simulink model "PUMA_fuzzy_dis"  (Simulink 8.9)
settings: Solver=ode15s  StartTime=0  StopTime=5  MaxStep=0.02  RelTol=1e-3  EnableMultiTasking=on
undefined symbols (not defined in the file): sfunxyz
libraries: aerolibutil x17, simulink x4, Fuzzy_Type2_Lib x3
(part 3 of 3)

== system PUMA_fuzzy_dis/3-Link PUMA Robot-Block /K or I matrix = fct (tau: torque, B, C, G, dteta) /B matrix/b412/I14 ==
  AI14 actual I14 : Constant  Value=0.00164
  Sum4 : Sum  Inputs=|++
  UI14 uncertainty added to I14 +- 0.0009 max : Constant  Value=UI14
  I14 : Outport
  wires:
  AI14 actual I14/1 -> Sum4/1
  UI14 uncertainty added to I14 +- 0.0009 max/1 -> Sum4/2
  Sum4/1 -> I14/1

== system PUMA_fuzzy_dis/3-Link PUMA Robot-Block /K or I matrix = fct (tau: torque, B, C, G, dteta) /B matrix/b412/I19 ==
  AI19 actual I19 : Constant  Value=0.0003
  Sum4 : Sum  Inputs=|++
  UI19 uncertainty added to I19 +- 0.0003 max : Constant  Value=UI19
  I19 : Outport
  wires:
  AI19 actual I19/1 -> Sum4/1
  UI19 uncertainty added to I19 +- 0.0003 max/1 -> Sum4/2
  Sum4/1 -> I19/1

== system PUMA_fuzzy_dis/3-Link PUMA Robot-Block /K or I matrix = fct (tau: torque, B, C, G, dteta) /B matrix/b412/I20 ==
  AI20 actual I20 : Constant  Value=-0.000202
  Sum4 : Sum  Inputs=|++
  UI20 uncertainty added to I20 +- 0.0008 max : Constant  Value=UI20
  I20 : Outport
  wires:
  AI20 actual I20/1 -> Sum4/1
  UI20 uncertainty added to I20 +- 0.0008 max/1 -> Sum4/2
  Sum4/1 -> I20/1

== system PUMA_fuzzy_dis/3-Link PUMA Robot-Block /K or I matrix = fct (tau: torque, B, C, G, dteta) /B matrix/b413/I14 ==
  AI14 actual I14 : Constant  Value=0.00164
  Sum4 : Sum  Inputs=|++
  UI14 uncertainty added to I14 +- 0.0009 max : Constant  Value=UI14
  I14 : Outport
  wires:
  AI14 actual I14/1 -> Sum4/1
  UI14 uncertainty added to I14 +- 0.0009 max/1 -> Sum4/2
  Sum4/1 -> I14/1

== system PUMA_fuzzy_dis/3-Link PUMA Robot-Block /K or I matrix = fct (tau: torque, B, C, G, dteta) /B matrix/b413/I19 ==
  AI19 actual I19 : Constant  Value=0.0003
  Sum4 : Sum  Inputs=|++
  UI19 uncertainty added to I19 +- 0.0003 max : Constant  Value=UI19
  I19 : Outport
  wires:
  AI19 actual I19/1 -> Sum4/1
  UI19 uncertainty added to I19 +- 0.0003 max/1 -> Sum4/2
  Sum4/1 -> I19/1

== system PUMA_fuzzy_dis/3-Link PUMA Robot-Block /K or I matrix = fct (tau: torque, B, C, G, dteta) /B matrix/b413/I20 ==
  AI20 actual I20 : Constant  Value=-0.000202
  Sum4 : Sum  Inputs=|++
  UI20 uncertainty added to I20 +- 0.0008 max : Constant  Value=UI20
  I20 : Outport
  wires:
  AI20 actual I20/1 -> Sum4/1
  UI20 uncertainty added to I20 +- 0.0008 max/1 -> Sum4/2
  Sum4/1 -> I20/1

== system PUMA_fuzzy_dis/3-Link PUMA Robot-Block /K or I matrix = fct (tau: torque, B, C, G, dteta) /B matrix/b415/I17 ==
  AI17 actual I17 : Constant  Value=0.000642
  Sum4 : Sum  Inputs=|++
  UI17 uncertainty added to I17 +- 0.0003 max : Constant  Value=UI17
  I17 : Outport
  wires:
  AI17 actual I17/1 -> Sum4/1
  UI17 uncertainty added to I17 +- 0.0003 max/1 -> Sum4/2
  Sum4/1 -> I17/1

== system PUMA_fuzzy_dis/3-Link PUMA Robot-Block /K or I matrix = fct (tau: torque, B, C, G, dteta) /B matrix/b415/I20 ==
  AI20 actual I20 : Constant  Value=-0.000202
  Sum4 : Sum  Inputs=|++
  UI20 uncertainty added to I20 +- 0.0008 max : Constant  Value=UI20
  I20 : Outport
  wires:
  AI20 actual I20/1 -> Sum4/1
  UI20 uncertainty added to I20 +- 0.0008 max/1 -> Sum4/2
  Sum4/1 -> I20/1

== system PUMA_fuzzy_dis/3-Link PUMA Robot-Block /K or I matrix = fct (tau: torque, B, C, G, dteta) /B matrix/b514/I17 ==
  AI17 actual I17 : Constant  Value=0.000642
  Sum4 : Sum  Inputs=|++
  UI17 uncertainty added to I17 +- 0.0003 max : Constant  Value=UI17
  I17 : Outport
  wires:
  AI17 actual I17/1 -> Sum4/1
  UI17 uncertainty added to I17 +- 0.0003 max/1 -> Sum4/2
  Sum4/1 -> I17/1

== system PUMA_fuzzy_dis/3-Link PUMA Robot-Block /K or I matrix = fct (tau: torque, B, C, G, dteta) /B matrix/b514/I20 ==
  AI20 actual I20 : Constant  Value=-0.000202
  Sum4 : Sum  Inputs=|++
  UI20 uncertainty added to I20 +- 0.0008 max : Constant  Value=UI20
  I20 : Outport
  wires:
  AI20 actual I20/1 -> Sum4/1
  UI20 uncertainty added to I20 +- 0.0008 max/1 -> Sum4/2
  Sum4/1 -> I20/1

== system PUMA_fuzzy_dis/3-Link PUMA Robot-Block /K or I matrix = fct (tau: torque, B, C, G, dteta) /C matrix/c12/I13 ==
  AI13 actual I13 : Constant  Value=-0.00379
  Sum4 : Sum  Inputs=|++
  UI13 uncertainty added to I13 +- 0.0009 max : Constant  Value=UI13
  I13 : Outport
  wires:
  AI13 actual I13/1 -> Sum4/1
  UI13 uncertainty added to I13 +- 0.0009 max/1 -> Sum4/2
  Sum4/1 -> I13/1

== system PUMA_fuzzy_dis/3-Link PUMA Robot-Block /K or I matrix = fct (tau: torque, B, C, G, dteta) /C matrix/c12/I18 ==
  AI18 actual I18 : Constant  Value=0.000431
  Sum4 : Sum  Inputs=|++
  UI18 uncertainty added to I18 +- 0.0003 max : Constant  Value=UI18
  I18 : Outport
  wires:
  AI18 actual I18/1 -> Sum4/1
  UI18 uncertainty added to I18 +- 0.0003 max/1 -> Sum4/2
  Sum4/1 -> I18/1

== system PUMA_fuzzy_dis/3-Link PUMA Robot-Block /K or I matrix = fct (tau: torque, B, C, G, dteta) /C matrix/c12/I4 ==
  AI4 actual I4 : Constant  Value=0.69
  Sum4 : Sum  Inputs=|++
  UI4 uncertainty added to I4 +- 0.02 max : Constant  Value=UI4
  I4 : Outport
  wires:
  AI4 actual I4/1 -> Sum4/1
  UI4 uncertainty added to I4 +- 0.02 max/1 -> Sum4/2
  Sum4/1 -> I4/1

== system PUMA_fuzzy_dis/3-Link PUMA Robot-Block /K or I matrix = fct (tau: torque, B, C, G, dteta) /C matrix/c12/I8 ==
  AI8 actual I8 : Constant  Value=-0.134
  Sum4 : Sum  Inputs=|++
  UI8 uncertainty added to I8 +- 0.014 max : Constant  Value=UI8
  I8 : Outport
  wires:
  AI8 actual I8/1 -> Sum4/1
  UI8 uncertainty added to I8 +- 0.014 max/1 -> Sum4/2
  Sum4/1 -> I8/1

== system PUMA_fuzzy_dis/3-Link PUMA Robot-Block /K or I matrix = fct (tau: torque, B, C, G, dteta) /C matrix/c12/I9 ==
  AI9 actual I9 : Constant  Value=0.0238
  Sum4 : Sum  Inputs=|++
  UI9 uncertainty added to I9 +- 0.014 max : Constant  Value=UI9
  I9 : Outport
  wires:
  AI9 actual I9/1 -> Sum4/1
  UI9 uncertainty added to I9 +- 0.014 max/1 -> Sum4/2
  Sum4/1 -> I9/1

== system PUMA_fuzzy_dis/3-Link PUMA Robot-Block /K or I matrix = fct (tau: torque, B, C, G, dteta) /C matrix/c13/I13 ==
  AI13 actual I13 : Constant  Value=-0.00379
  Sum4 : Sum  Inputs=|++
  UI13 uncertainty added to I13 +- 0.0009 max : Constant  Value=UI13
  I13 : Outport
  wires:
  AI13 actual I13/1 -> Sum4/1
  UI13 uncertainty added to I13 +- 0.0009 max/1 -> Sum4/2
  Sum4/1 -> I13/1

== system PUMA_fuzzy_dis/3-Link PUMA Robot-Block /K or I matrix = fct (tau: torque, B, C, G, dteta) /C matrix/c13/I18 ==
  AI18 actual I18 : Constant  Value=0.000431
  Sum4 : Sum  Inputs=|++
  UI18 uncertainty added to I18 +- 0.0003 max : Constant  Value=UI18
  I18 : Outport
  wires:
  AI18 actual I18/1 -> Sum4/1
  UI18 uncertainty added to I18 +- 0.0003 max/1 -> Sum4/2
  Sum4/1 -> I18/1

== system PUMA_fuzzy_dis/3-Link PUMA Robot-Block /K or I matrix = fct (tau: torque, B, C, G, dteta) /C matrix/c13/I8 ==
  AI8 actual I8 : Constant  Value=-0.134
  Sum4 : Sum  Inputs=|++
  UI8 uncertainty added to I8 +- 0.014 max : Constant  Value=UI8
  I8 : Outport
  wires:
  AI8 actual I8/1 -> Sum4/1
  UI8 uncertainty added to I8 +- 0.014 max/1 -> Sum4/2
  Sum4/1 -> I8/1

== system PUMA_fuzzy_dis/3-Link PUMA Robot-Block /K or I matrix = fct (tau: torque, B, C, G, dteta) /C matrix/c21/I10 ==
  AI10 actual I10 : Constant  Value=-0.0213
  Sum4 : Sum  Inputs=|++
  UI10 uncertainty added to I10 +- 0.022 max : Constant  Value=UI10
  I10 : Outport
  wires:
  AI10 actual I10/1 -> Sum4/1
  UI10 uncertainty added to I10 +- 0.022 max/1 -> Sum4/2
  Sum4/1 -> I10/1

== system PUMA_fuzzy_dis/3-Link PUMA Robot-Block /K or I matrix = fct (tau: torque, B, C, G, dteta) /C matrix/c21/I11 ==
  AI11 actual I11 : Constant  Value=-0.0142
  Sum4 : Sum  Inputs=|++
  UI11 uncertainty added to I11 +- 0.007 max : Constant  Value=UI11
  I11 : Outport
  wires:
  AI11 actual I11/1 -> Sum4/1
  UI11 uncertainty added to I11 +- 0.007 max/1 -> Sum4/2
  Sum4/1 -> I11/1

== system PUMA_fuzzy_dis/3-Link PUMA Robot-Block /K or I matrix = fct (tau: torque, B, C, G, dteta) /C matrix/c21/I12 ==
  AI12 actual I12 : Constant  Value=-0.011
  Sum4 : Sum  Inputs=|++
  UI12 uncertainty added to I12 +- 0.0011 max : Constant  Value=UI12
  I12 : Outport
  wires:
  AI12 actual I12/1 -> Sum4/1
  UI12 uncertainty added to I12 +- 0.0011 max/1 -> Sum4/2
  Sum4/1 -> I12/1

== system PUMA_fuzzy_dis/3-Link PUMA Robot-Block /K or I matrix = fct (tau: torque, B, C, G, dteta) /C matrix/c21/I15 ==
  AI15 actual I15 : Constant  Value=0.00125
  Sum4 : Sum  Inputs=|++
  UI15 uncertainty added to I15 +- 0.0003 max : Constant  Value=UI15
  I15 : Outport
  wires:
  AI15 actual I15/1 -> Sum4/1
  UI15 uncertainty added to I15 +- 0.0003 max/1 -> Sum4/2
  Sum4/1 -> I15/1

== system PUMA_fuzzy_dis/3-Link PUMA Robot-Block /K or I matrix = fct (tau: torque, B, C, G, dteta) /C matrix/c21/I16 ==
  AI16 actual I16 : Constant  Value=0.00124
  Sum4 : Sum  Inputs=|++
  UI16 uncertainty added to I16 +- 0.0003 max : Constant  Value=UI16
  I16 : Outport
  wires:
  AI16 actual I16/1 -> Sum4/1
  UI16 uncertainty added to I16 +- 0.0003 max/1 -> Sum4/2
  Sum4/1 -> I16/1

== system PUMA_fuzzy_dis/3-Link PUMA Robot-Block /K or I matrix = fct (tau: torque, B, C, G, dteta) /C matrix/c21/I21 ==
  AI21 actual I21 : Constant  Value=-0.0001
  Sum4 : Sum  Inputs=|++
  UI21 uncertainty added to I21 +- 0.0006 max : Constant  Value=UI21
  I21 : Outport
  wires:
  AI21 actual I21/1 -> Sum4/1
  UI21 uncertainty added to I21 +- 0.0006 max/1 -> Sum4/2
  Sum4/1 -> I21/1

== system PUMA_fuzzy_dis/3-Link PUMA Robot-Block /K or I matrix = fct (tau: torque, B, C, G, dteta) /C matrix/c21/I22 ==
  AI22 actual I22 : Constant  Value=-0.000058
  Sum4 : Sum  Inputs=|++
  UI22 uncertainty added to I22 +- 0.000015 max : Constant  Value=UI22
  I22 : Outport
  wires:
  AI22 actual I22/1 -> Sum4/1
  UI22 uncertainty added to I22 +- 0.000015 max/1 -> Sum4/2
  Sum4/1 -> I22/1

== system PUMA_fuzzy_dis/3-Link PUMA Robot-Block /K or I matrix = fct (tau: torque, B, C, G, dteta) /C matrix/c21/I3 ==
  AI3 actual I3 : Constant  Value=1.38
  Sum4 : Sum  Inputs=|++
  UI3 uncertainty added to I3 +- 0.05 max : Constant  Value=UI3
  I3 : Outport
  wires:
  AI3 actual I3/1 -> Sum4/1
  UI3 uncertainty added to I3 +- 0.05 max/1 -> Sum4/2
  Sum4/1 -> I3/1

== system PUMA_fuzzy_dis/3-Link PUMA Robot-Block /K or I matrix = fct (tau: torque, B, C, G, dteta) /C matrix/c21/I5 ==
  AI5 actual I5 : Constant  Value=0.372
  Sum4 : Sum  Inputs=|++
  UI5 uncertainty added to I5 +- 0.05 max : Constant  Value=UI5
  I5 : Outport
  wires:
  AI5 actual I5/1 -> Sum4/1
  UI5 uncertainty added to I5 +- 0.05 max/1 -> Sum4/2
  Sum4/1 -> I5/1

== system PUMA_fuzzy_dis/3-Link PUMA Robot-Block /K or I matrix = fct (tau: torque, B, C, G, dteta) /C matrix/c21/I7 ==
  AI7 actual I7 : Constant  Value=0.298
  Sum4 : Sum  Inputs=|++
  UI7 uncertainty added to I7 +- 0.029 max : Constant  Value=UI7
  I7 : Outport
  wires:
  AI7 actual I7/1 -> Sum4/1
  UI7 uncertainty added to I7 +- 0.029 max/1 -> Sum4/2
  Sum4/1 -> I7/1

== system PUMA_fuzzy_dis/3-Link PUMA Robot-Block /K or I matrix = fct (tau: torque, B, C, G, dteta) /C matrix/c23/I12 ==
  AI12 actual I12 : Constant  Value=-0.011
  Sum4 : Sum  Inputs=|++
  UI12 uncertainty added to I12 +- 0.0011 max : Constant  Value=UI12
  I12 : Outport
  wires:
  AI12 actual I12/1 -> Sum4/1
  UI12 uncertainty added to I12 +- 0.0011 max/1 -> Sum4/2
  Sum4/1 -> I12/1

== system PUMA_fuzzy_dis/3-Link PUMA Robot-Block /K or I matrix = fct (tau: torque, B, C, G, dteta) /C matrix/c23/I16 ==
  AI16 actual I16 : Constant  Value=0.00124
  Sum4 : Sum  Inputs=|++
  UI16 uncertainty added to I16 +- 0.0003 max : Constant  Value=UI16
  I16 : Outport
  wires:
  AI16 actual I16/1 -> Sum4/1
  UI16 uncertainty added to I16 +- 0.0003 max/1 -> Sum4/2
  Sum4/1 -> I16/1

== system PUMA_fuzzy_dis/3-Link PUMA Robot-Block /K or I matrix = fct (tau: torque, B, C, G, dteta) /C matrix/c23/I5 ==
  AI5 actual I5 : Constant  Value=0.372
  Sum4 : Sum  Inputs=|++
  UI5 uncertainty added to I5 +- 0.05 max : Constant  Value=UI5
  I5 : Outport
  wires:
  AI5 actual I5/1 -> Sum4/1
  UI5 uncertainty added to I5 +- 0.05 max/1 -> Sum4/2
  Sum4/1 -> I5/1

== system PUMA_fuzzy_dis/3-Link PUMA Robot-Block /K or I matrix = fct (tau: torque, B, C, G, dteta) /C matrix/c31/I10 ==
  AI10 actual I10 : Constant  Value=-0.0213
  Sum4 : Sum  Inputs=|++
  UI10 uncertainty added to I10 +- 0.022 max : Constant  Value=UI10
  I10 : Outport
  wires:
  AI10 actual I10/1 -> Sum4/1
  UI10 uncertainty added to I10 +- 0.022 max/1 -> Sum4/2
  Sum4/1 -> I10/1

== system PUMA_fuzzy_dis/3-Link PUMA Robot-Block /K or I matrix = fct (tau: torque, B, C, G, dteta) /C matrix/c31/I12 ==
  AI12 actual I12 : Constant  Value=-0.011
  Sum4 : Sum  Inputs=|++
  UI12 uncertainty added to I12 +- 0.0011 max : Constant  Value=UI12
  I12 : Outport
  wires:
  AI12 actual I12/1 -> Sum4/1
  UI12 uncertainty added to I12 +- 0.0011 max/1 -> Sum4/2
  Sum4/1 -> I12/1

== system PUMA_fuzzy_dis/3-Link PUMA Robot-Block /K or I matrix = fct (tau: torque, B, C, G, dteta) /C matrix/c31/I15 ==
  AI15 actual I15 : Constant  Value=0.00125
  Sum4 : Sum  Inputs=|++
  UI15 uncertainty added to I15 +- 0.0003 max : Constant  Value=UI15
  I15 : Outport
  wires:
  AI15 actual I15/1 -> Sum4/1
  UI15 uncertainty added to I15 +- 0.0003 max/1 -> Sum4/2
  Sum4/1 -> I15/1

== system PUMA_fuzzy_dis/3-Link PUMA Robot-Block /K or I matrix = fct (tau: torque, B, C, G, dteta) /C matrix/c31/I16 ==
  AI16 actual I16 : Constant  Value=0.00124
  Sum4 : Sum  Inputs=|++
  UI16 uncertainty added to I16 +- 0.0003 max : Constant  Value=UI16
  I16 : Outport
  wires:
  AI16 actual I16/1 -> Sum4/1
  UI16 uncertainty added to I16 +- 0.0003 max/1 -> Sum4/2
  Sum4/1 -> I16/1

== system PUMA_fuzzy_dis/3-Link PUMA Robot-Block /K or I matrix = fct (tau: torque, B, C, G, dteta) /C matrix/c31/I21 ==
  AI21 actual I21 : Constant  Value=-0.0001
  Sum4 : Sum  Inputs=|++
  UI21 uncertainty added to I21 +- 0.0006 max : Constant  Value=UI21
  I21 : Outport
  wires:
  AI21 actual I21/1 -> Sum4/1
  UI21 uncertainty added to I21 +- 0.0006 max/1 -> Sum4/2
  Sum4/1 -> I21/1

== system PUMA_fuzzy_dis/3-Link PUMA Robot-Block /K or I matrix = fct (tau: torque, B, C, G, dteta) /C matrix/c31/I22 ==
  AI22 actual I22 : Constant  Value=-0.000058
  Sum4 : Sum  Inputs=|++
  UI22 uncertainty added to I22 +- 0.000015 max : Constant  Value=UI22
  I22 : Outport
  wires:
  AI22 actual I22/1 -> Sum4/1
  UI22 uncertainty added to I22 +- 0.000015 max/1 -> Sum4/2
  Sum4/1 -> I22/1

== system PUMA_fuzzy_dis/3-Link PUMA Robot-Block /K or I matrix = fct (tau: torque, B, C, G, dteta) /C matrix/c31/I5 ==
  AI5 actual I5 : Constant  Value=0.372
  Sum4 : Sum  Inputs=|++
  UI5 uncertainty added to I5 +- 0.05 max : Constant  Value=UI5
  I5 : Outport
  wires:
  AI5 actual I5/1 -> Sum4/1
  UI5 uncertainty added to I5 +- 0.05 max/1 -> Sum4/2
  Sum4/1 -> I5/1

== system PUMA_fuzzy_dis/3-Link PUMA Robot-Block /K or I matrix = fct (tau: torque, B, C, G, dteta) /C matrix/c31/I7 ==
  AI7 actual I7 : Constant  Value=0.298
  Sum4 : Sum  Inputs=|++
  UI7 uncertainty added to I7 +- 0.029 max : Constant  Value=UI7
  I7 : Outport
  wires:
  AI7 actual I7/1 -> Sum4/1
  UI7 uncertainty added to I7 +- 0.029 max/1 -> Sum4/2
  Sum4/1 -> I7/1

== system PUMA_fuzzy_dis/3-Link PUMA Robot-Block /K or I matrix = fct (tau: torque, B, C, G, dteta) /C matrix/c32/I12 ==
  AI12 actual I12 : Constant  Value=-0.011
  Sum4 : Sum  Inputs=|++
  UI12 uncertainty added to I12 +- 0.0011 max : Constant  Value=UI12
  I12 : Outport
  wires:
  AI12 actual I12/1 -> Sum4/1
  UI12 uncertainty added to I12 +- 0.0011 max/1 -> Sum4/2
  Sum4/1 -> I12/1

== system PUMA_fuzzy_dis/3-Link PUMA Robot-Block /K or I matrix = fct (tau: torque, B, C, G, dteta) /C matrix/c32/I16 ==
  AI16 actual I16 : Constant  Value=0.00124
  Sum4 : Sum  Inputs=|++
  UI16 uncertainty added to I16 +- 0.0003 max : Constant  Value=UI16
  I16 : Outport
  wires:
  AI16 actual I16/1 -> Sum4/1
  UI16 uncertainty added to I16 +- 0.0003 max/1 -> Sum4/2
  Sum4/1 -> I16/1

== system PUMA_fuzzy_dis/3-Link PUMA Robot-Block /K or I matrix = fct (tau: torque, B, C, G, dteta) /C matrix/c32/I5 ==
  AI5 actual I5 : Constant  Value=0.372
  Sum4 : Sum  Inputs=|++
  UI5 uncertainty added to I5 +- 0.05 max : Constant  Value=UI5
  I5 : Outport
  wires:
  AI5 actual I5/1 -> Sum4/1
  UI5 uncertainty added to I5 +- 0.05 max/1 -> Sum4/2
  Sum4/1 -> I5/1

== system PUMA_fuzzy_dis/3-Link PUMA Robot-Block /K or I matrix = fct (tau: torque, B, C, G, dteta) /C matrix/c51/I15 ==
  AI15 actual I15 : Constant  Value=0.00125
  Sum4 : Sum  Inputs=|++
  UI15 uncertainty added to I15 +- 0.0003 max : Constant  Value=UI15
  I15 : Outport
  wires:
  AI15 actual I15/1 -> Sum4/1
  UI15 uncertainty added to I15 +- 0.0003 max/1 -> Sum4/2
  Sum4/1 -> I15/1

== system PUMA_fuzzy_dis/3-Link PUMA Robot-Block /K or I matrix = fct (tau: torque, B, C, G, dteta) /C matrix/c51/I16 ==
  AI16 actual I16 : Constant  Value=0.00124
  Sum4 : Sum  Inputs=|++
  UI16 uncertainty added to I16 +- 0.0003 max : Constant  Value=UI16
  I16 : Outport
  wires:
  AI16 actual I16/1 -> Sum4/1
  UI16 uncertainty added to I16 +- 0.0003 max/1 -> Sum4/2
  Sum4/1 -> I16/1

== system PUMA_fuzzy_dis/3-Link PUMA Robot-Block /K or I matrix = fct (tau: torque, B, C, G, dteta) /C matrix/c51/I22 ==
  AI22 actual I22 : Constant  Value=-0.000058
  Sum4 : Sum  Inputs=|++
  UI22 uncertainty added to I22 +- 0.000015 max : Constant  Value=UI22
  I22 : Outport
  wires:
  AI22 actual I22/1 -> Sum4/1
  UI22 uncertainty added to I22 +- 0.000015 max/1 -> Sum4/2
  Sum4/1 -> I22/1

== system PUMA_fuzzy_dis/3-Link PUMA Robot-Block /K or I matrix = fct (tau: torque, B, C, G, dteta) /C matrix/c52/I16 ==
  AI16 actual I16 : Constant  Value=0.00124
  Sum4 : Sum  Inputs=|++
  UI16 uncertainty added to I16 +- 0.0003 max : Constant  Value=UI16
  I16 : Outport
  wires:
  AI16 actual I16/1 -> Sum4/1
  UI16 uncertainty added to I16 +- 0.0003 max/1 -> Sum4/2
  Sum4/1 -> I16/1

== system PUMA_fuzzy_dis/3-Link PUMA Robot-Block /K or I matrix = fct (tau: torque, B, C, G, dteta) /C matrix/c52/I22 ==
  AI22 actual I22 : Constant  Value=-0.000058
  Sum4 : Sum  Inputs=|++
  UI22 uncertainty added to I22 +- 0.000015 max : Constant  Value=UI22
  I22 : Outport
  wires:
  AI22 actual I22/1 -> Sum4/1
  UI22 uncertainty added to I22 +- 0.000015 max/1 -> Sum4/2
  Sum4/1 -> I22/1

== system PUMA_fuzzy_dis/3-Link PUMA Robot-Block /K or I matrix = fct (tau: torque, B, C, G, dteta) /Gravity matrix/g2 term/g1 ==
  G1 : Constant  Value=-37.2
  Sum4 : Sum  Inputs=|++
  UG1 uncertainty added to G1 +- 0.5 max : Constant  Value=UG1
  g1 : Outport
  wires:
  G1/1 -> Sum4/1
  UG1 uncertainty added to G1 +- 0.5 max/1 -> Sum4/2
  Sum4/1 -> g1/1

== system PUMA_fuzzy_dis/3-Link PUMA Robot-Block /K or I matrix = fct (tau: torque, B, C, G, dteta) /Gravity matrix/g2 term/g2 ==
  G2 : Constant  Value=-8.44
  Sum4 : Sum  Inputs=|++
  UG2 uncertainty added to G2 +- 0.2 max : Constant  Value=UG2
  g2 : Outport
  wires:
  G2/1 -> Sum4/1
  UG2 uncertainty added to G2 +- 0.2 max/1 -> Sum4/2
  Sum4/1 -> g2/1

== system PUMA_fuzzy_dis/3-Link PUMA Robot-Block /K or I matrix = fct (tau: torque, B, C, G, dteta) /Gravity matrix/g2 term/g3 ==
  G3 : Constant  Value=1.02
  Sum4 : Sum  Inputs=|++
  UG3 uncertainty added to G3 +- 0.5 max : Constant  Value=UG3
  g3 : Outport
  wires:
  G3/1 -> Sum4/1
  UG3 uncertainty added to G3 +- 0.5 max/1 -> Sum4/2
  Sum4/1 -> g3/1

== system PUMA_fuzzy_dis/3-Link PUMA Robot-Block /K or I matrix = fct (tau: torque, B, C, G, dteta) /Gravity matrix/g2 term/g4 ==
  G4 : Constant  Value=0.249
  Sum4 : Sum  Inputs=|++
  UG4 uncertainty added to G4 +- 0.025 max : Constant  Value=UG4
  g4 : Outport
  wires:
  G4/1 -> Sum4/1
  UG4 uncertainty added to G4 +- 0.025 max/1 -> Sum4/2
  Sum4/1 -> g4/1

== system PUMA_fuzzy_dis/3-Link PUMA Robot-Block /K or I matrix = fct (tau: torque, B, C, G, dteta) /Gravity matrix/g2 term/g5 ==
  G5 : Constant  Value=-0.0282
  Sum4 : Sum  Inputs=|++
  UG5 uncertainty added to G5 +- 0.0056 max : Constant  Value=UG5
  g5 : Outport
  wires:
  G5/1 -> Sum4/1
  UG5 uncertainty added to G5 +- 0.0056 max/1 -> Sum4/2
  Sum4/1 -> g5/1

== system PUMA_fuzzy_dis/3-Link PUMA Robot-Block /K or I matrix = fct (tau: torque, B, C, G, dteta) /Gravity matrix/g3 term/g2 ==
  G2 : Constant  Value=-8.44
  Sum4 : Sum  Inputs=|++
  UG2 uncertainty added to G2 +- 0.2 max : Constant  Value=UG2
  g2 : Outport
  wires:
  G2/1 -> Sum4/1
  UG2 uncertainty added to G2 +- 0.2 max/1 -> Sum4/2
  Sum4/1 -> g2/1

== system PUMA_fuzzy_dis/3-Link PUMA Robot-Block /K or I matrix = fct (tau: torque, B, C, G, dteta) /Gravity matrix/g3 term/g4 ==
  G4 : Constant  Value=0.249
  Sum4 : Sum  Inputs=|++
  UG4 uncertainty added to G4 +- 0.025 max : Constant  Value=UG4
  g4 : Outport
  wires:
  G4/1 -> Sum4/1
  UG4 uncertainty added to G4 +- 0.025 max/1 -> Sum4/2
  Sum4/1 -> g4/1

== system PUMA_fuzzy_dis/3-Link PUMA Robot-Block /K or I matrix = fct (tau: torque, B, C, G, dteta) /Gravity matrix/g3 term/g5 ==
  G5 : Constant  Value=-0.0282
  Sum4 : Sum  Inputs=|++
  UG5 uncertainty added to G5 +- 0.0056 max : Constant  Value=UG5
  g5 : Outport
  wires:
  G5/1 -> Sum4/1
  UG5 uncertainty added to G5 +- 0.0056 max/1 -> Sum4/2
  Sum4/1 -> g5/1

== system PUMA_fuzzy_dis/3-Link PUMA Robot-Block /K or I matrix = fct (tau: torque, B, C, G, dteta) /Gravity matrix/g5 term/g5 ==
  G5 : Constant  Value=-0.0282
  Sum4 : Sum  Inputs=|++
  UG5 uncertainty added to G5 +- 0.0056 max : Constant  Value=UG5
  g5 : Outport
  wires:
  G5/1 -> Sum4/1
  UG5 uncertainty added to G5 +- 0.0056 max/1 -> Sum4/2
  Sum4/1 -> g5/1

== matlab function Kinematics of 3 DOF PUMA ==
  data: px output double; py output double; pz output double; teta1 input double; teta2 input double; teta3 input double; desiredteta1 input double; desiredteta2 input double; desiredteta3 input double; desiredx output double; desiredy output double; desiredz output double
function [px,py,pz,desiredx,desiredy,desiredz] = fcn(teta1,teta2,teta3,desiredteta1,desiredteta2,desiredteta3)
% This block supports an embeddable subset of the MATLAB language.
% this block finds the end-effector position given the angles

px = cos(teta1)*[-0.4331*sin(teta2+teta3)-0.0203*cos(teta2+teta3)+0.4318*cos(teta2)]+0.0934*sin(teta1);
py = sin(teta1)*[-0.4331*sin(teta2+teta3)-0.0203*cos(teta2+teta3)+0.4318*cos(teta2)]-0.0934*sin(teta1);
pz = -0.4331*cos(teta2+teta3)+0.0203*sin(teta2+teta3)-0.4318*sin(teta2);


desiredx = cos(desiredteta1)*[-0.4331*sin(desiredteta2+desiredteta3)-0.0203*cos(desiredteta2+desiredteta3)+0.4318*cos(desiredteta2)]+0.0934*sin(desiredteta1);
desiredy = sin(desiredteta1)*[-0.4331*sin(desiredteta2+desiredteta3)-0.0203*cos(desiredteta2+desiredteta3)+0.4318*cos(desiredteta2)]-0.0934*sin(desiredteta1);
desiredz = -0.4331*cos(desiredteta2+desiredteta3)+0.0203*sin(desiredteta2+desiredteta3)-0.4318*sin(desiredteta2);

== matlab function 3-Link PUMA Robot-Block /6x6 inverse matrix calculator ==
  data: a11 output double; a12 output double; a13 output double; a14 output double; a15 output double; a16 output double; a21 output double; a22 output double; a23 output double; a24 output double; a25 output double; a26 output double; a31 output double; a32 output double; a33 output double; b11 input double; b12 input double; b13 input double; b14 input double; b15 input double; b16 input double; b21 input double; b22 input double; b23 input double; b24 input double; b25 input double; b26 input double; b31 input double; b32 input double; b33 input double; b34 input double; b35 input double; b36 input double; b41 input double; b42 input double; b43 input double; b44 input double; b45 input double; b46 input double; b51 input double; b52 input double; b53 input double; b54 input double; b55 input double; b56 input double; b61 input double; b62 input double; b63 input double; b64 input double; b65 input double; b66 input double; a34 output double; a35 output double; a36 output double; a41 output double; a42 output double; a43 output double; a44 output double; a45 output double; a46 output double; a51 output double; a52 output double; a53 output double; a54 output double; a55 output double; a56 output double; a61 output double; a62 output double; a63 output double; a64 output double; a65 output double; a66 output double
function [a11, a12, a13, a14,a15,a16,a21, a22, a23, a24,a25,a26,a31, a32, a33, a34,a35,a36,a41, a42, a43, a44,a45,a46,a51, a52, a53, a54,a55,a56,a61, a62, a63, a64,a65,a66] = fcn(b11, b12, b13, b14,b15,b16,b21, b22, b23, b24,b25,b26,b31, b32, b33, b34,b35,b36,b41, b42, b43, b44,b45,b46,b51, b52, b53, b54,b55,b56,b61, b62, b63, b64,b65,b66)
% This block supports an embeddable subset of the MATLAB language.
% this block finds the inverse of a 6x6 matrix

B=[b11, b12, b13, b14,b15,b16;b21, b22, b23, b24,b25,b26;b31, b32, b33, b34,b35,b36;b41, b42, b43, b44,b45,b46;b51, b52, b53, b54,b55,b56;b61, b62, b63, b64,b65,b66];
A=inv(B);

a11=A(1,1);
a12=A(1,2);
a13=A(1,3);
a14=A(1,4);
a15=A(1,5);
a16=A(1,6);

a21=A(2,1);
a22=A(2,2);
a23=A(2,3);
a24=A(2,4);
a25=A(2,5);
a26=A(2,6);

a31=A(3,1);
a32=A(3,2);
a33=A(3,3);
a34=A(3,4);
a35=A(3,5);
a36=A(3,6);

a41=A(4,1);
a42=A(4,2);
a43=A(4,3);
a44=A(4,4);
a45=A(4,5);
a46=A(4,6);

a51=A(5,1);
a52=A(5,2);
a53=A(5,3);
a54=A(5,4);
a55=A(5,5);
a56=A(5,6);

a61=A(6,1);
a62=A(6,2);
a63=A(6,3);
a64=A(6,4);
a65=A(6,5);
a66=A(6,6);

== matlab function Fuzzy Controller/last three joints controller to keep zero position ==
  data: teta1 input double; teta2 input double; teta3 input double; dteta1 input double; dteta2 input double; dteta3 input double; T4 output double; T5 output double; T6 output double
function [T4,T5,T6] = fcn(teta1,teta2,teta3,dteta1,dteta2,dteta3)
% This block supports an embeddable subset of the MATLAB language.
% this block finds the end-effector position given the angles
%berdus



% values of the control needed to keep the last three joints zero 
I14=.00164;
I15=.00125;
I16=.00124;
I17=.000642;
I18=.000431;
I19=.0003;
I20=-.000202;
I22=-.000058;
g5=-.0282;

b412=-(I14*sin(teta2+teta3)+I19*sin(teta2+teta3)+I20*sin(teta2+teta3));
b413=-((I20*+I14+I19)*sin(teta2+teta3));

c51=-(-sin(teta2+teta3)*cos(teta2+teta3)+I15*sin(teta2+teta3)*cos(teta2+teta3)+I16*cos(teta2)*cos(teta2+teta3)+I22*cos(teta2+teta3)^2);
c52=-(I16*cos(teta3)+I22);
G5=g5*sin(teta2+teta3);

T4 = b412*dteta1*dteta2 + b413*dteta1*dteta3;
T5 = c51*dteta1^2 + c52*dteta2^2 + g5;
T6 = 0;
